simulink model "lab7_6"  (R2018b)
settings: Solver=FixedStepDiscrete  StartTime=0.0  StopTime=1000000  FixedStep=1  RelTol=1e-3
libraries: hdlsllib x2, simulink x1
settings Model: Creator=mllax8  LastModifiedBy=mllax8

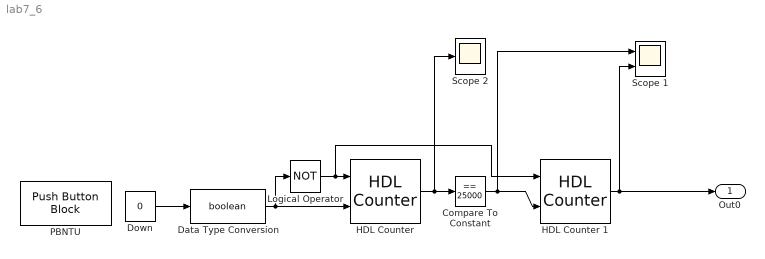
== system lab7_6 ==
  Compare To Constant : simulink/Logic and Bit Operations/Compare To Constant  relop===  const=25000  OutDataTypeStr=boolean
  Data Type Conversion : DataTypeConversion  OutDataTypeStr=boolean
  Down : Constant  Value=0
  "HDL Counter " : hdlsllib/Sources/HDL Counter  CountType=Count limited  CountInit=0  CountStep=1  CountMax=100000  CountFromType=Initial value  CountFrom=0  CountResetPort=on  CountLoadPort=off  CountEnbPort=on  CountDirPort=off  CountDataType=Unsigned  CountWordLen=18  CountFracLen=0  CountSampTime=1
      settings: SourceProductBaseCode=HD
  HDL Counter 1 : hdlsllib/Sources/HDL Counter  CountType=Free running  CountInit=0  CountStep=1  CountMax=25  CountFromType=Initial value  CountFrom=0  CountResetPort=on  CountLoadPort=off  CountEnbPort=on  CountDirPort=off  CountDataType=Unsigned  CountWordLen=1  CountFracLen=0  CountSampTime=1
      settings: SourceProductBaseCode=HD
  Logical Operator : Logic  Operator=NOT  AllPortsSameDT=off  OutDataTypeStr=boolean
  PBNTU : PushButtonBlock  WebBlockId=91
  Scope 1 : Scope  NumInputPorts=2
  Scope 2 : Scope
  Out0 : Outport
  wires:
  "HDL Counter "/1 -> Scope 2/1, Compare To Constant/1
  Compare To Constant/1 -> HDL Counter 1/2, Scope 1/1
  Logical Operator/1 -> HDL Counter 1/1, "HDL Counter "/1
  Data Type Conversion/1 -> "HDL Counter "/2, Logical Operator/1
  HDL Counter 1/1 -> Scope 1/2, Out0/1
  Down/1 -> Data Type Conversion/1
